simulink model "mbdo_centroidal"  (Simulink 9.0)
settings: Solver=ode45  StartTime=0.0  StopTime=10  MaxStep=0.001  RelTol=1e-3  EnableMultiTasking=on
InitFcn:
  | mbdoParams
StartFcn:
  | mbdoParams
undefined symbols (not defined in the file or in its folder): computeVcross, Gain, Ic
undefined symbols (not defined in the file): inputForce, Kdang, Kdlin, Kpang, Kplin
settings Model: SuppressorTable=22 serialization::archive 11 0 6 0 0 0 11 0  Creator=mfocchi  LastModifiedBy=nikhil
settings DataIOCC: LimitDataPoints=on  SignalLoggingSaveFormat=ModelDataLogs
settings OptimizationCC: ExpressionDepthLimit=2147483647  InitFltsAndDblsToZero=on
settings DebuggingCC: SolverPrmCheckMsg=warning  FcnCallInpInsideContextMsg=warning  StateNameClashWarn=warning
settings GRTTargetCC: CombineOutputUpdateFcns=off  GRTInterface=on

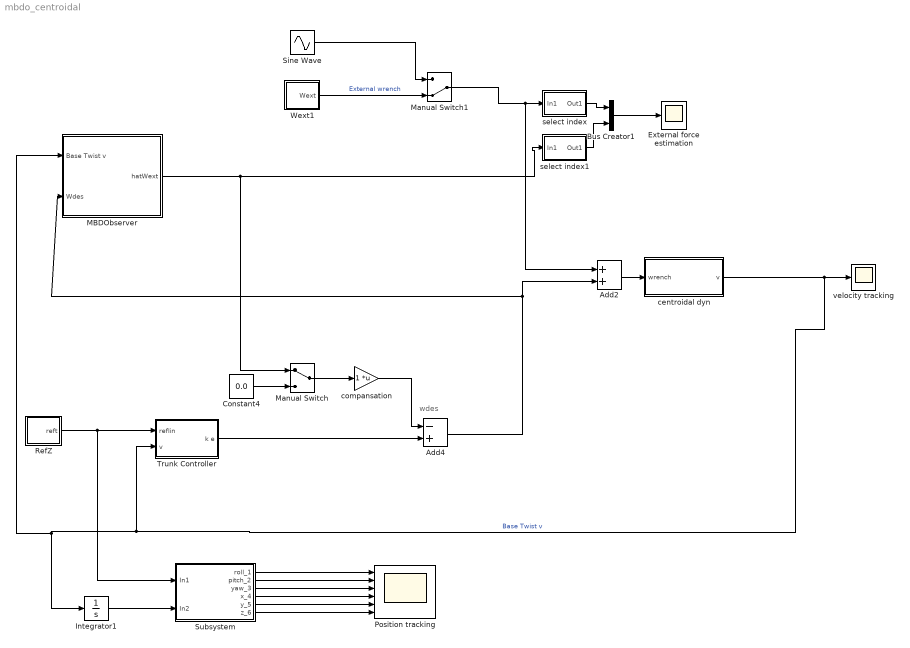
== system mbdo_centroidal ==
  note: wdes
  Add2 : Sum
  Add4 : Sum  Inputs=-+
  Bus Creator1 : BusCreator  Inputs=2
  Constant4 : Constant  Value=0.0
  External force estimation : Scope
  Integrator1 : Integrator
  MBDObserver : Subsystem
  Manual Switch : ManualSwitch
  Manual Switch1 : ManualSwitch  CurrentSetting=0
  Position tracking : Scope  NumInputPorts=6
  RefZ : Subsystem  mask{input=6, value=0.2}
  Sine Wave : Sin  Amplitude=100  Frequency=2*pi*5  SampleTime=0
  Subsystem : Subsystem
  Trunk Controller : Subsystem
  Wext1 : Subsystem  mask{input=inputForce, fext=200, step_time=3}
  centroidal dyn : Subsystem
  compansation : Gain  Multiplication=Matrix(K*u)
  select index : Subsystem  mask{input=inputForce}
  "select index1 " : Subsystem  mask{input=inputForce}
  velocity tracking : Scope
  wires:
  Add2/1 -> centroidal dyn/1(wrench)
  Manual Switch/1 -> compansation/1
  Constant4/1 -> Manual Switch/2
  centroidal dyn/1(v) -> velocity tracking/1, Trunk Controller/2(v), MBDObserver/1(Base Twist v), Integrator1/1  "Base Twist v"
  RefZ/1(reft) -> Trunk Controller/1(reflin), Subsystem/1(In1)
  Trunk Controller/1(k e) -> Add4/2
  Bus Creator1/1 -> External force estimation/1
  select index/1(Out1) -> Bus Creator1/1
  "select index1 "/1(Out1) -> Bus Creator1/2
  compansation/1 -> Add4/1
  Manual Switch1/1 -> Add2/1, select index/1(In1)
  Wext1/1(Wext) -> Manual Switch1/2  "External wrench"
  Sine Wave/1 -> Manual Switch1/1
  Integrator1/1 -> Subsystem/2(In2)
  Subsystem/1(roll_1) -> Position tracking/1
  Subsystem/2(pitch_2) -> Position tracking/2
  Subsystem/3(yaw_3) -> Position tracking/3
  Subsystem/4(x_4) -> Position tracking/4
  Subsystem/5(y_5) -> Position tracking/5
  Subsystem/6(z_6) -> Position tracking/6
  MBDObserver/1("hatWext ") -> Manual Switch/1, "select index1 "/1(In1)
  Add4/1 -> MBDObserver/2(Wdes), Add2/2

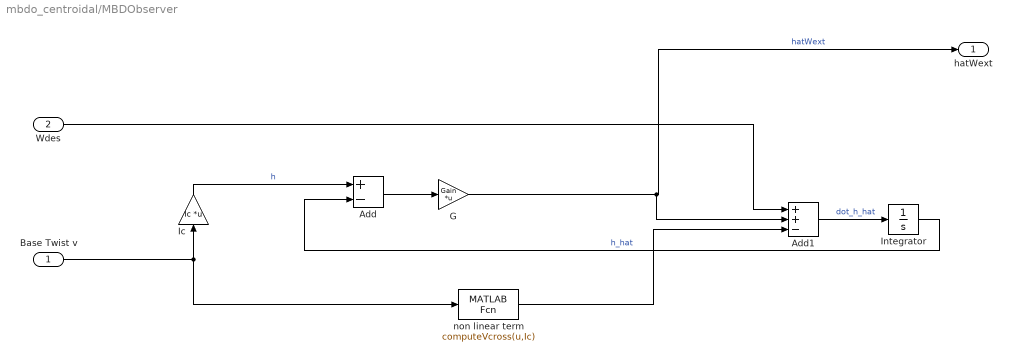
== system mbdo_centroidal/MBDObserver ==
  Base Twist v : Inport
  Wdes : Inport  Port=2
  Add : Sum  Inputs=+-
  Add1 : Sum  Inputs=++-
  G : Gain  Gain=Gain  Multiplication=Matrix(K*u)
  Ic : Gain  Gain=Ic  Multiplication=Matrix(K*u)
  Integrator : Integrator
  non linear term : MATLABFcn  MATLABFcn=computeVcross(u,Ic)
  "hatWext " : Outport
  wires:
  G/1 -> Add1/2, "hatWext "/1  "hatWext"
  Wdes/1 -> Add1/1
  Base Twist v/1 -> non linear term/1, Ic/1
  Add/1 -> G/1
  Add1/1 -> Integrator/1  "dot_h_hat"
  Ic/1 -> Add/1  "h"
  Integrator/1 -> Add/2  "h_hat"
  non linear term/1 -> Add1/3

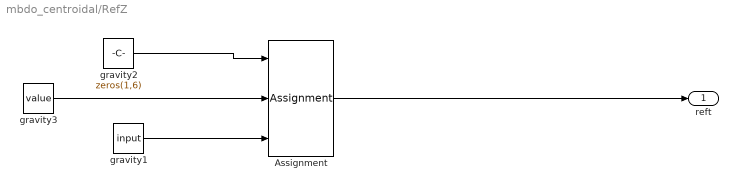
== system mbdo_centroidal/RefZ ==
  Assignment : Assignment  IndexOptions=Index vector (port)  Indices=1  OutputSizes=1
  gravity1 : Constant  Value=input
  gravity2 : Constant  Value=zeros(1,6)
  gravity3 : Constant  Value=value
  reft : Outport
  wires:
  gravity3/1 -> Assignment/2
  Assignment/1 -> reft/1
  gravity1/1 -> Assignment/3
  gravity2/1 -> Assignment/1

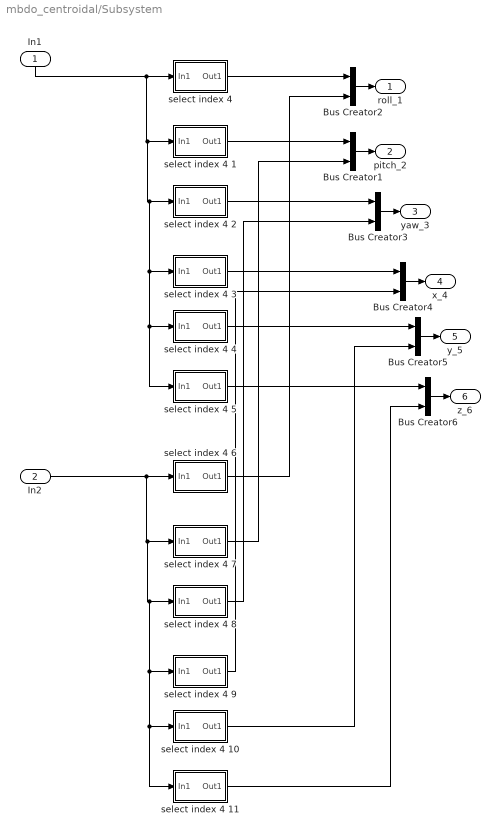
== system mbdo_centroidal/Subsystem ==
  In1 : Inport
  In2 : Inport  Port=2
  Bus Creator{1..6} (6 alike) : BusCreator  Inputs=2
  "select index 4 " : Subsystem  mask{input=1}
  select index 4 1 : Subsystem  mask{input=2}
  select index 4 10 : Subsystem  mask{input=5}
  select index 4 11 : Subsystem  mask{input=6}
  select index 4 2 : Subsystem  mask{input=3}
  select index 4 3 : Subsystem  mask{input=4}
  select index 4 4 : Subsystem  mask{input=5}
  select index 4 5 : Subsystem  mask{input=6}
  select index 4 6 : Subsystem  mask{input=1}
  select index 4 7 : Subsystem  mask{input=2}
  select index 4 8 : Subsystem  mask{input=3}
  select index 4 9 : Subsystem  mask{input=4}
  roll_1 : Outport
  pitch_2 : Outport  Port=2
  yaw_3 : Outport  Port=3
  x_4 : Outport  Port=4
  y_5 : Outport  Port=5
  z_6 : Outport  Port=6
  wires:
  Bus Creator2/1 -> roll_1/1
  "select index 4 "/1(Out1) -> Bus Creator2/1
  In1/1 -> select index 4 5/1(In1), select index 4 4/1(In1), select index 4 3/1(In1), select index 4 2/1(In1), select index 4 1/1(In1), "select index 4 "/1(In1)
  In2/1 -> select index 4 11/1(In1), select index 4 10/1(In1), select index 4 9/1(In1), select index 4 8/1(In1), select index 4 7/1(In1), select index 4 6/1(In1)
  select index 4 6/1(Out1) -> Bus Creator2/2
  select index 4 7/1(Out1) -> Bus Creator1/2
  select index 4 1/1(Out1) -> Bus Creator1/1
  Bus Creator1/1 -> pitch_2/1
  Bus Creator3/1 -> yaw_3/1
  select index 4 8/1(Out1) -> Bus Creator3/2
  select index 4 9/1(Out1) -> Bus Creator4/2
  Bus Creator4/1 -> x_4/1
  Bus Creator5/1 -> y_5/1
  select index 4 10/1(Out1) -> Bus Creator5/2
  select index 4 11/1(Out1) -> Bus Creator6/2
  Bus Creator6/1 -> z_6/1
  select index 4 2/1(Out1) -> Bus Creator3/1
  select index 4 3/1(Out1) -> Bus Creator4/1
  select index 4 4/1(Out1) -> Bus Creator5/1
  select index 4 5/1(Out1) -> Bus Creator6/1

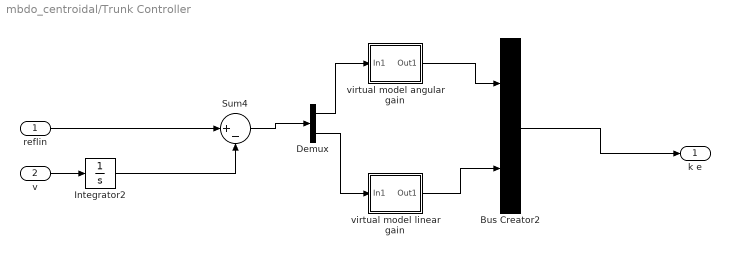
== system mbdo_centroidal/Trunk Controller ==
  reflin : Inport
  v : Inport  Port=2
  Bus Creator2 : BusCreator  Inputs=2
  Demux : Demux  Outputs=2
  Integrator2 : Integrator  InitialCondition=0.0
  Sum4 : Sum  Inputs=|+-
  virtual model angular gain : Subsystem  mask{stiffness=Kpang, damping=Kdang}
  virtual model linear gain : Subsystem  mask{stiffness=Kplin, damping=Kdlin}
  k e : Outport
  wires:
  Demux/2 -> virtual model linear gain/1(In1)
  Sum4/1 -> Demux/1
  Demux/1 -> virtual model angular gain/1(In1)
  virtual model linear gain/1(Out1) -> Bus Creator2/2
  virtual model angular gain/1(Out1) -> Bus Creator2/1
  Integrator2/1 -> Sum4/2
  v/1 -> Integrator2/1
  Bus Creator2/1 -> k e/1
  reflin/1 -> Sum4/1

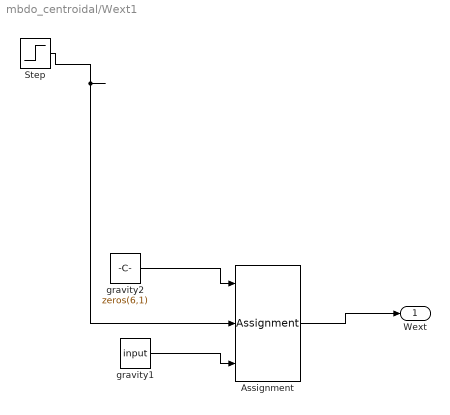
== system mbdo_centroidal/Wext1 ==
  Assignment : Assignment  IndexOptions=Index vector (port)  Indices=1  OutputSizes=1
  Step : Step  Time=step_time  After=fext  SampleTime=0
  gravity1 : Constant  Value=input
  gravity2 : Constant  Value=zeros(6,1)
  Wext : Outport
  wires:
  Step/1 -> Assignment/2
  gravity2/1 -> Assignment/1
  gravity1/1 -> Assignment/3
  Assignment/1 -> Wext/1

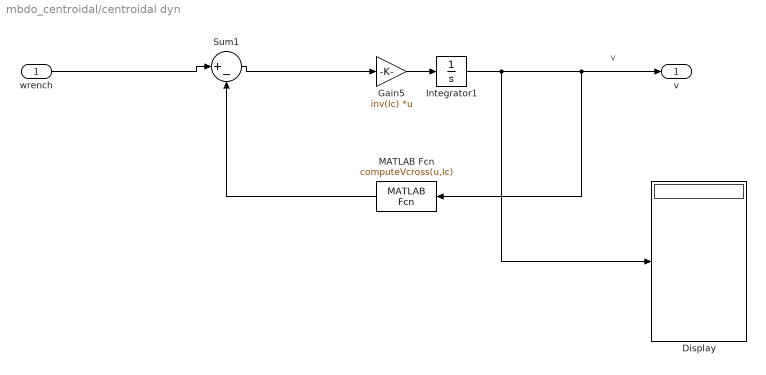
== system mbdo_centroidal/centroidal dyn ==
  note: v
  wrench : Inport
  Display : Display
  Gain5 : Gain  Gain=inv(Ic)  Multiplication=Matrix(K*u)
  Integrator1 : Integrator  InitialCondition=0.0
  MATLAB Fcn : MATLABFcn  MATLABFcn=computeVcross(u,Ic)
  Sum1 : Sum  Inputs=|+-
  v : Outport
  wires:
  MATLAB Fcn/1 -> Sum1/2
  wrench/1 -> Sum1/1
  Integrator1/1 -> v/1, MATLAB Fcn/1, Display/1
  Gain5/1 -> Integrator1/1
  Sum1/1 -> Gain5/1

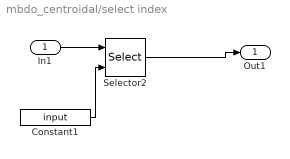
== system mbdo_centroidal/select index ==
  In1 : Inport
  Constant1 : Constant  Value=input
  Selector2 : Selector  InputPortWidth=6  IndexOptions=Index vector (port)  Indices=[1 ]  OutputSizes=1
  Out1 : Outport
  wires:
  Constant1/1 -> Selector2/2
  In1/1 -> Selector2/1
  Selector2/1 -> Out1/1

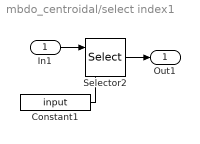
== system mbdo_centroidal/select index1  ==
  In1 : Inport
  Constant1 : Constant  Value=input
  Selector2 : Selector  InputPortWidth=6  IndexOptions=Index vector (port)  Indices=[1 ]  OutputSizes=1
  Out1 : Outport
  wires:
  Selector2/1 -> Out1/1
  In1/1 -> Selector2/1
  Constant1/1 -> Selector2/2

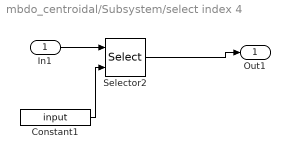
== system mbdo_centroidal/Subsystem/select index 4  ==
  In1 : Inport
  Constant1 : Constant  Value=input
  Selector2 : Selector  InputPortWidth=6  IndexOptions=Index vector (port)  Indices=[1 ]  OutputSizes=1
  Out1 : Outport
  wires:
  Selector2/1 -> Out1/1
  In1/1 -> Selector2/1
  Constant1/1 -> Selector2/2

== system mbdo_centroidal/Subsystem/select index 4 1 ==
  In1 : Inport
  Constant1 : Constant  Value=input
  Selector2 : Selector  InputPortWidth=6  IndexOptions=Index vector (port)  Indices=[1 ]  OutputSizes=1
  Out1 : Outport
  wires:
  Constant1/1 -> Selector2/2
  In1/1 -> Selector2/1
  Selector2/1 -> Out1/1

== system mbdo_centroidal/Subsystem/select index 4 10 ==
  In1 : Inport
  Constant1 : Constant  Value=input
  Selector2 : Selector  InputPortWidth=6  IndexOptions=Index vector (port)  Indices=[1 ]  OutputSizes=1
  Out1 : Outport
  wires:
  Selector2/1 -> Out1/1
  In1/1 -> Selector2/1
  Constant1/1 -> Selector2/2

== system mbdo_centroidal/Subsystem/select index 4 11 ==
  In1 : Inport
  Constant1 : Constant  Value=input
  Selector2 : Selector  InputPortWidth=6  IndexOptions=Index vector (port)  Indices=[1 ]  OutputSizes=1
  Out1 : Outport
  wires:
  Constant1/1 -> Selector2/2
  In1/1 -> Selector2/1
  Selector2/1 -> Out1/1

== system mbdo_centroidal/Subsystem/select index 4 2 ==
  In1 : Inport
  Constant1 : Constant  Value=input
  Selector2 : Selector  InputPortWidth=6  IndexOptions=Index vector (port)  Indices=[1 ]  OutputSizes=1
  Out1 : Outport
  wires:
  Selector2/1 -> Out1/1
  In1/1 -> Selector2/1
  Constant1/1 -> Selector2/2

== system mbdo_centroidal/Subsystem/select index 4 3 ==
  In1 : Inport
  Constant1 : Constant  Value=input
  Selector2 : Selector  InputPortWidth=6  IndexOptions=Index vector (port)  Indices=[1 ]  OutputSizes=1
  Out1 : Outport
  wires:
  Constant1/1 -> Selector2/2
  In1/1 -> Selector2/1
  Selector2/1 -> Out1/1

== system mbdo_centroidal/Subsystem/select index 4 4 ==
  In1 : Inport
  Constant1 : Constant  Value=input
  Selector2 : Selector  InputPortWidth=6  IndexOptions=Index vector (port)  Indices=[1 ]  OutputSizes=1
  Out1 : Outport
  wires:
  Selector2/1 -> Out1/1
  In1/1 -> Selector2/1
  Constant1/1 -> Selector2/2

== system mbdo_centroidal/Subsystem/select index 4 5 ==
  In1 : Inport
  Constant1 : Constant  Value=input
  Selector2 : Selector  InputPortWidth=6  IndexOptions=Index vector (port)  Indices=[1 ]  OutputSizes=1
  Out1 : Outport
  wires:
  Constant1/1 -> Selector2/2
  In1/1 -> Selector2/1
  Selector2/1 -> Out1/1

== system mbdo_centroidal/Subsystem/select index 4 6 ==
  In1 : Inport
  Constant1 : Constant  Value=input
  Selector2 : Selector  InputPortWidth=6  IndexOptions=Index vector (port)  Indices=[1 ]  OutputSizes=1
  Out1 : Outport
  wires:
  Selector2/1 -> Out1/1
  In1/1 -> Selector2/1
  Constant1/1 -> Selector2/2

== system mbdo_centroidal/Subsystem/select index 4 7 ==
  In1 : Inport
  Constant1 : Constant  Value=input
  Selector2 : Selector  InputPortWidth=6  IndexOptions=Index vector (port)  Indices=[1 ]  OutputSizes=1
  Out1 : Outport
  wires:
  Constant1/1 -> Selector2/2
  In1/1 -> Selector2/1
  Selector2/1 -> Out1/1

== system mbdo_centroidal/Subsystem/select index 4 8 ==
  In1 : Inport
  Constant1 : Constant  Value=input
  Selector2 : Selector  InputPortWidth=6  IndexOptions=Index vector (port)  Indices=[1 ]  OutputSizes=1
  Out1 : Outport
  wires:
  Selector2/1 -> Out1/1
  In1/1 -> Selector2/1
  Constant1/1 -> Selector2/2

== system mbdo_centroidal/Subsystem/select index 4 9 ==
  In1 : Inport
  Constant1 : Constant  Value=input
  Selector2 : Selector  InputPortWidth=6  IndexOptions=Index vector (port)  Indices=[1 ]  OutputSizes=1
  Out1 : Outport
  wires:
  Constant1/1 -> Selector2/2
  In1/1 -> Selector2/1
  Selector2/1 -> Out1/1

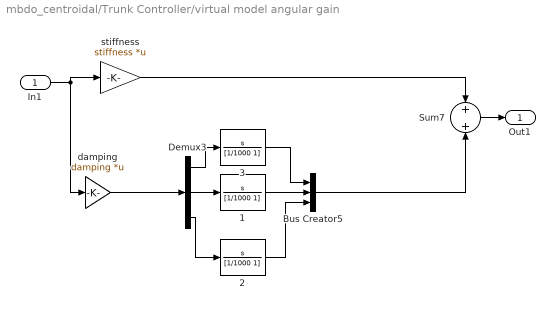
== system mbdo_centroidal/Trunk Controller/virtual model angular gain ==
  In1 : Inport
  " 1" : TransferFcn  Numerator=[1 0]  Denominator=[1/1000 1]
  " 2" : TransferFcn  Numerator=[1 0]  Denominator=[1/1000 1]
  " 3" : TransferFcn  Numerator=[1 0]  Denominator=[1/1000 1]
  Bus Creator5 : BusCreator  Inputs=3
  Demux3 : Demux  Outputs=3
  Sum7 : Sum  Inputs=+|+
  damping : Gain  Gain=damping  Multiplication=Matrix(K*u)
  stiffness : Gain  Gain=stiffness  Multiplication=Matrix(K*u)
  Out1 : Outport
  wires:
  Bus Creator5/1 -> Sum7/2
  damping/1 -> Demux3/1
  " 2"/1 -> Bus Creator5/3
  " 1"/1 -> Bus Creator5/2
  " 3"/1 -> Bus Creator5/1
  Demux3/3 -> " 2"/1
  Demux3/2 -> " 1"/1
  Demux3/1 -> " 3"/1
  Sum7/1 -> Out1/1
  In1/1 -> stiffness/1, damping/1
  stiffness/1 -> Sum7/1

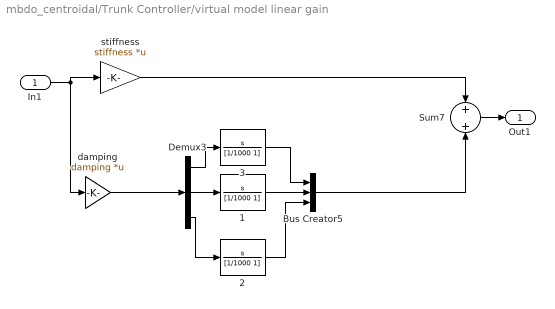
== system mbdo_centroidal/Trunk Controller/virtual model linear gain ==
  In1 : Inport
  " 1" : TransferFcn  Numerator=[1 0]  Denominator=[1/1000 1]
  " 2" : TransferFcn  Numerator=[1 0]  Denominator=[1/1000 1]
  " 3" : TransferFcn  Numerator=[1 0]  Denominator=[1/1000 1]
  Bus Creator5 : BusCreator  Inputs=3
  Demux3 : Demux  Outputs=3
  Sum7 : Sum  Inputs=+|+
  damping : Gain  Gain=damping  Multiplication=Matrix(K*u)
  stiffness : Gain  Gain=stiffness  Multiplication=Matrix(K*u)
  Out1 : Outport
  wires:
  stiffness/1 -> Sum7/1
  In1/1 -> damping/1, stiffness/1
  Sum7/1 -> Out1/1
  Demux3/1 -> " 3"/1
  Demux3/2 -> " 1"/1
  Demux3/3 -> " 2"/1
  " 3"/1 -> Bus Creator5/1
  " 1"/1 -> Bus Creator5/2
  " 2"/1 -> Bus Creator5/3
  damping/1 -> Demux3/1
  Bus Creator5/1 -> Sum7/2
